simulink model "case1"  (R2024b)
settings: Solver=FixedStepAuto  StartTime=0  StopTime=1  FixedStep=1e-7  RelTol=1e-3
values from neighbouring files (symbols this model uses):
  SG_D_1_D = 0.01056    [IEEE9_case_parameters.m]    (also in case1_parameters.m; case2_parameters.m; case3_parameters.m; case4_parameters.m)
  SG_D_1_EnableSaturation = 0    [IEEE9_case_parameters.m]    (also in case1_parameters.m; case2_parameters.m; case3_parameters.m; case4_parameters.m)
  SG_D_1_f0 = 60    [IEEE9_case_parameters.m]    (also in case1_parameters.m; case2_parameters.m; case3_parameters.m; case4_parameters.m)
  SG_D_1_H = 7.5    [IEEE9_case_parameters.m]    (also in case1_parameters.m; case2_parameters.m; case3_parameters.m; case4_parameters.m)
  SG_D_1_K_A = 20    [IEEE9_case_parameters.m]    (also in case1_parameters.m; case2_parameters.m; case3_parameters.m; case4_parameters.m)
  SG_D_1_K_E = 1.000000e+1    (= 10)    [IEEE9_case_parameters.m]    (also in case1_parameters.m; case2_parameters.m; case3_parameters.m; case4_parameters.m)
  SG_D_1_K_F = 2.363    [IEEE9_case_parameters.m]    (also in case1_parameters.m; case2_parameters.m; case3_parameters.m; case4_parameters.m)
  SG_D_1_K_s = 0.5    [IEEE9_case_parameters.m]    (also in case1_parameters.m = 5; case2_parameters.m = 5; case3_parameters.m = 5; case4_parameters.m = 5)
  SG_D_1_R_a = 0.001088    [IEEE9_case_parameters.m]    (also in case1_parameters.m; case2_parameters.m; case3_parameters.m; case4_parameters.m)
  SG_D_1_S_A = 1    [IEEE9_case_parameters.m]    (also in case1_parameters.m; case2_parameters.m; case3_parameters.m; case4_parameters.m)
  SG_D_1_S_B = 0.103    [IEEE9_case_parameters.m]    (also in case1_parameters.m; case2_parameters.m; case3_parameters.m; case4_parameters.m)
  SG_D_1_S_N = 10.659857    [IEEE9_case_parameters.m]    (also in case1_parameters.m; case2_parameters.m; case3_parameters.m; case4_parameters.m)
  SG_D_1_SpeedPara = 200    [IEEE9_case_parameters.m]    (also in case1_parameters.m; case2_parameters.m; case3_parameters.m; case4_parameters.m)
  SG_D_1_T_0 = 0.720173    [IEEE9_case_parameters.m]    (also in case1_parameters.m = 0.755522; case2_parameters.m = 0.808931; case3_parameters.m = 0.869402; case4_parameters.m = 0.729316)
  SG_D_1_T_1 = 0.3    [IEEE9_case_parameters.m]    (also in case1_parameters.m; case2_parameters.m; case3_parameters.m; case4_parameters.m)
  SG_D_1_T_2 = 0.05    [IEEE9_case_parameters.m]    (also in case1_parameters.m; case2_parameters.m; case3_parameters.m; case4_parameters.m)
  SG_D_1_T_3 = 0.02    [IEEE9_case_parameters.m]    (also in case1_parameters.m; case2_parameters.m; case3_parameters.m; case4_parameters.m)
  SG_D_1_T_4 = 0.005    [IEEE9_case_parameters.m]    (also in case1_parameters.m; case2_parameters.m; case3_parameters.m; case4_parameters.m)
  SG_D_1_T_A = 0.02    [IEEE9_case_parameters.m]    (also in case1_parameters.m; case2_parameters.m; case3_parameters.m; case4_parameters.m)
  SG_D_1_T_dd = 8.000000e+0    (= 8)    [IEEE9_case_parameters.m]    (also in case1_parameters.m; case2_parameters.m; case3_parameters.m; case4_parameters.m)
  SG_D_1_T_ddd = 0.04    [IEEE9_case_parameters.m]    (also in case1_parameters.m; case2_parameters.m; case3_parameters.m; case4_parameters.m)
  SG_D_1_T_E = 0.314    [IEEE9_case_parameters.m]    (also in case1_parameters.m; case2_parameters.m; case3_parameters.m; case4_parameters.m)
  SG_D_1_T_F = 0.35    [IEEE9_case_parameters.m]    (also in case1_parameters.m; case2_parameters.m; case3_parameters.m; case4_parameters.m)
  SG_D_1_T_qd = 0.8    [IEEE9_case_parameters.m]    (also in case1_parameters.m; case2_parameters.m; case3_parameters.m; case4_parameters.m)
  SG_D_1_T_qdd = 0.02    [IEEE9_case_parameters.m]    (also in case1_parameters.m; case2_parameters.m; case3_parameters.m; case4_parameters.m)
  SG_D_1_T_speed = 0.1    [IEEE9_case_parameters.m]    (also in case1_parameters.m = 200; case2_parameters.m = 200; case3_parameters.m = 200; case4_parameters.m = 200)
  SG_D_1_T_w = 0.5    [IEEE9_case_parameters.m]    (also in case1_parameters.m; case2_parameters.m; case3_parameters.m; case4_parameters.m)
  SG_D_1_V_ref = 1.990276    [IEEE9_case_parameters.m]    (also in case1_parameters.m = 2.042296; case2_parameters.m = 2.051388; case3_parameters.m = 2.089584; case4_parameters.m = 2.01845)
  SG_D_1_w_ref = 376.991118    [IEEE9_case_parameters.m]    (also in case1_parameters.m; case2_parameters.m; case3_parameters.m; case4_parameters.m)
  SG_D_1_wb = 6.000000e+1    (= 60)    [IEEE9_case_parameters.m]    (also in case1_parameters.m; case2_parameters.m; case3_parameters.m; case4_parameters.m)
  SG_D_1_x_d = 1.9    [IEEE9_case_parameters.m]    (also in case1_parameters.m; case2_parameters.m; case3_parameters.m; case4_parameters.m)
  SG_D_1_x_dd = 0.302    [IEEE9_case_parameters.m]    (also in case1_parameters.m; case2_parameters.m; case3_parameters.m; case4_parameters.m)
  SG_D_1_x_ddd = 0.204    [IEEE9_case_parameters.m]    (also in case1_parameters.m; case2_parameters.m; case3_parameters.m; case4_parameters.m)
  SG_D_1_x_l = 0.05    [IEEE9_case_parameters.m]    (also in case1_parameters.m; case2_parameters.m; case3_parameters.m; case4_parameters.m)
  SG_D_1_x_q = 1.3    [IEEE9_case_parameters.m]    (also in case1_parameters.m; case2_parameters.m; case3_parameters.m; case4_parameters.m)
  SG_D_1_x_qd = 0.5    [IEEE9_case_parameters.m]    (also in case1_parameters.m; case2_parameters.m; case3_parameters.m; case4_parameters.m)
  SG_D_1_x_qdd = 0.3    [IEEE9_case_parameters.m]    (also in case1_parameters.m; case2_parameters.m; case3_parameters.m; case4_parameters.m)
  SG_D_2_D = 0.02    [IEEE9_case_parameters.m]    (also in case1_parameters.m; case2_parameters.m; case3_parameters.m; case4_parameters.m)
  SG_D_2_EnableSaturation = 0    [IEEE9_case_parameters.m]    (also in case1_parameters.m; case2_parameters.m; case3_parameters.m; case4_parameters.m)
  SG_D_2_f0 = 60    [IEEE9_case_parameters.m]    (also in case1_parameters.m; case2_parameters.m; case3_parameters.m; case4_parameters.m)
  SG_D_2_H = 8.000000e+0    (= 8)    [IEEE9_case_parameters.m]    (also in case1_parameters.m; case2_parameters.m; case3_parameters.m; case4_parameters.m)
  SG_D_2_K_A = 20    [IEEE9_case_parameters.m]    (also in case1_parameters.m; case2_parameters.m; case3_parameters.m; case4_parameters.m)
  SG_D_2_K_E = 1.000000e+1    (= 10)    [IEEE9_case_parameters.m]    (also in case1_parameters.m; case2_parameters.m; case3_parameters.m; case4_parameters.m)
  SG_D_2_K_F = 2.363    [IEEE9_case_parameters.m]    (also in case1_parameters.m; case2_parameters.m; case3_parameters.m; case4_parameters.m)
  SG_D_2_K_s = 0.5    [IEEE9_case_parameters.m]    (also in case1_parameters.m = 4; case2_parameters.m = 4; case3_parameters.m = 4; case4_parameters.m = 4)
  SG_D_2_R_a = 0.001088    [IEEE9_case_parameters.m]    (also in case1_parameters.m; case2_parameters.m; case3_parameters.m; case4_parameters.m)
  SG_D_2_S_A = 1    [IEEE9_case_parameters.m]    (also in case1_parameters.m; case2_parameters.m; case3_parameters.m; case4_parameters.m)
  SG_D_2_S_B = 0.103    [IEEE9_case_parameters.m]    (also in case1_parameters.m; case2_parameters.m; case3_parameters.m; case4_parameters.m)
  SG_D_2_S_N = 10.659857    [IEEE9_case_parameters.m]    (also in case1_parameters.m; case2_parameters.m; case3_parameters.m; case4_parameters.m)
  SG_D_2_SpeedPara = 200    [IEEE9_case_parameters.m]    (also in case1_parameters.m; case2_parameters.m; case3_parameters.m; case4_parameters.m)
  SG_D_2_T_0 = 1.632913    [IEEE9_case_parameters.m]    (also in case1_parameters.m = 1.632925; case2_parameters.m = 1.632915; case3_parameters.m = 1.632914; case4_parameters.m = 1.632927)
  SG_D_2_T_1 = 0.2    [IEEE9_case_parameters.m]    (also in case1_parameters.m; case2_parameters.m; case3_parameters.m; case4_parameters.m)
  SG_D_2_T_2 = 0.05    [IEEE9_case_parameters.m]    (also in case1_parameters.m; case2_parameters.m; case3_parameters.m; case4_parameters.m)
  SG_D_2_T_3 = 0.02    [IEEE9_case_parameters.m]    (also in case1_parameters.m; case2_parameters.m; case3_parameters.m; case4_parameters.m)
  SG_D_2_T_4 = 0.005    [IEEE9_case_parameters.m]    (also in case1_parameters.m; case2_parameters.m; case3_parameters.m; case4_parameters.m)
  SG_D_2_T_A = 0.02    [IEEE9_case_parameters.m]    (also in case1_parameters.m; case2_parameters.m; case3_parameters.m; case4_parameters.m)
  SG_D_2_T_dd = 7.9    [IEEE9_case_parameters.m]    (also in case1_parameters.m; case2_parameters.m; case3_parameters.m; case4_parameters.m)
  SG_D_2_T_ddd = 0.04    [IEEE9_case_parameters.m]    (also in case1_parameters.m; case2_parameters.m; case3_parameters.m; case4_parameters.m)
  SG_D_2_T_E = 0.314    [IEEE9_case_parameters.m]    (also in case1_parameters.m; case2_parameters.m; case3_parameters.m; case4_parameters.m)
  SG_D_2_T_F = 0.35    [IEEE9_case_parameters.m]    (also in case1_parameters.m; case2_parameters.m; case3_parameters.m; case4_parameters.m)
  SG_D_2_T_qd = 0.8    [IEEE9_case_parameters.m]    (also in case1_parameters.m; case2_parameters.m; case3_parameters.m; case4_parameters.m)
  SG_D_2_T_qdd = 0.015    [IEEE9_case_parameters.m]    (also in case1_parameters.m; case2_parameters.m; case3_parameters.m; case4_parameters.m)
  SG_D_2_T_speed = 0.1    [IEEE9_case_parameters.m]    (also in case1_parameters.m = 150; case2_parameters.m = 150; case3_parameters.m = 150; case4_parameters.m = 150)
  SG_D_2_T_w = 0.35    [IEEE9_case_parameters.m]    (also in case1_parameters.m; case2_parameters.m; case3_parameters.m; case4_parameters.m)
  SG_D_2_V_ref = 2.58547    [IEEE9_case_parameters.m]    (also in case1_parameters.m = 2.597896; case2_parameters.m = 2.587136; case3_parameters.m = 2.586042; case4_parameters.m = 2.599679)
  SG_D_2_w_ref = 376.991118    [IEEE9_case_parameters.m]    (also in case1_parameters.m; case2_parameters.m; case3_parameters.m; case4_parameters.m)
  SG_D_2_wb = 6.000000e+1    (= 60)    [IEEE9_case_parameters.m]    (also in case1_parameters.m; case2_parameters.m; case3_parameters.m; case4_parameters.m)
  SG_D_2_x_d = 1.8    [IEEE9_case_parameters.m]    (also in case1_parameters.m; case2_parameters.m; case3_parameters.m; case4_parameters.m)
  SG_D_2_x_dd = 0.302    [IEEE9_case_parameters.m]    (also in case1_parameters.m; case2_parameters.m; case3_parameters.m; case4_parameters.m)
  SG_D_2_x_ddd = 0.204    [IEEE9_case_parameters.m]    (also in case1_parameters.m; case2_parameters.m; case3_parameters.m; case4_parameters.m)
  SG_D_2_x_l = 0.05    [IEEE9_case_parameters.m]    (also in case1_parameters.m; case2_parameters.m; case3_parameters.m; case4_parameters.m)
  SG_D_2_x_q = 1.25    [IEEE9_case_parameters.m]    (also in case1_parameters.m; case2_parameters.m; case3_parameters.m; case4_parameters.m)
  SG_D_2_x_qd = 0.5    [IEEE9_case_parameters.m]    (also in case1_parameters.m; case2_parameters.m; case3_parameters.m; case4_parameters.m)
  SG_D_2_x_qdd = 0.3    [IEEE9_case_parameters.m]    (also in case1_parameters.m; case2_parameters.m; case3_parameters.m; case4_parameters.m)
  SG_D_3_D = 0.02    [IEEE9_case_parameters.m]    (also in case1_parameters.m; case2_parameters.m; case3_parameters.m; case4_parameters.m)
  SG_D_3_EnableSaturation = 0    [IEEE9_case_parameters.m]    (also in case1_parameters.m; case2_parameters.m; case3_parameters.m; case4_parameters.m)
  SG_D_3_f0 = 60    [IEEE9_case_parameters.m]    (also in case1_parameters.m; case2_parameters.m; case3_parameters.m; case4_parameters.m)
  SG_D_3_H = 7.7    [IEEE9_case_parameters.m]    (also in case1_parameters.m; case2_parameters.m; case3_parameters.m; case4_parameters.m)
  SG_D_3_K_A = 20    [IEEE9_case_parameters.m]    (also in case1_parameters.m; case2_parameters.m; case3_parameters.m; case4_parameters.m)
  SG_D_3_K_E = 1.000000e+1    (= 10)    [IEEE9_case_parameters.m]    (also in case1_parameters.m; case2_parameters.m; case3_parameters.m; case4_parameters.m)
  SG_D_3_K_F = 2.363    [IEEE9_case_parameters.m]    (also in case1_parameters.m; case2_parameters.m; case3_parameters.m; case4_parameters.m)
  SG_D_3_K_s = 0.2    [IEEE9_case_parameters.m]    (also in case1_parameters.m = 2; case2_parameters.m = 2; case3_parameters.m = 2; case4_parameters.m = 2)
  SG_D_3_R_a = 0.001088    [IEEE9_case_parameters.m]    (also in case1_parameters.m; case2_parameters.m; case3_parameters.m; case4_parameters.m)
  SG_D_3_S_A = 1    [IEEE9_case_parameters.m]    (also in case1_parameters.m; case2_parameters.m; case3_parameters.m; case4_parameters.m)
  SG_D_3_S_B = 0.103    [IEEE9_case_parameters.m]    (also in case1_parameters.m; case2_parameters.m; case3_parameters.m; case4_parameters.m)
  SG_D_3_S_N = 10.659857    [IEEE9_case_parameters.m]    (also in case1_parameters.m; case2_parameters.m; case3_parameters.m; case4_parameters.m)
  SG_D_3_SpeedPara = 200    [IEEE9_case_parameters.m]    (also in case1_parameters.m; case2_parameters.m; case3_parameters.m; case4_parameters.m)
  SG_D_3_T_0 = 0.850788    [IEEE9_case_parameters.m]    (also in case1_parameters.m = 0.850786; case2_parameters.m = 0.850787; case3_parameters.m; case4_parameters.m = 0.850786)
  SG_D_3_T_1 = 0.2    [IEEE9_case_parameters.m]    (also in case1_parameters.m; case2_parameters.m; case3_parameters.m; case4_parameters.m)
  SG_D_3_T_2 = 0.05    [IEEE9_case_parameters.m]    (also in case1_parameters.m; case2_parameters.m; case3_parameters.m; case4_parameters.m)
  SG_D_3_T_3 = 0.02    [IEEE9_case_parameters.m]    (also in case1_parameters.m; case2_parameters.m; case3_parameters.m; case4_parameters.m)
  SG_D_3_T_4 = 0.005    [IEEE9_case_parameters.m]    (also in case1_parameters.m; case2_parameters.m; case3_parameters.m; case4_parameters.m)
  SG_D_3_T_A = 0.02    [IEEE9_case_parameters.m]    (also in case1_parameters.m; case2_parameters.m; case3_parameters.m; case4_parameters.m)
  SG_D_3_T_dd = 8.1    [IEEE9_case_parameters.m]    (also in case1_parameters.m; case2_parameters.m; case3_parameters.m; case4_parameters.m)
  SG_D_3_T_ddd = 0.04    [IEEE9_case_parameters.m]    (also in case1_parameters.m; case2_parameters.m; case3_parameters.m; case4_parameters.m)
  SG_D_3_T_E = 0.314    [IEEE9_case_parameters.m]    (also in case1_parameters.m; case2_parameters.m; case3_parameters.m; case4_parameters.m)
  SG_D_3_T_F = 0.35    [IEEE9_case_parameters.m]    (also in case1_parameters.m; case2_parameters.m; case3_parameters.m; case4_parameters.m)
  SG_D_3_T_qd = 0.8    [IEEE9_case_parameters.m]    (also in case1_parameters.m; case2_parameters.m; case3_parameters.m; case4_parameters.m)
  SG_D_3_T_qdd = 0.015    [IEEE9_case_parameters.m]    (also in case1_parameters.m; case2_parameters.m; case3_parameters.m; case4_parameters.m)
  SG_D_3_T_speed = 0.1    [IEEE9_case_parameters.m]    (also in case1_parameters.m = 180; case2_parameters.m = 180; case3_parameters.m = 180; case4_parameters.m = 180)
  SG_D_3_T_w = 0.4    [IEEE9_case_parameters.m]    (also in case1_parameters.m; case2_parameters.m; case3_parameters.m; case4_parameters.m)
  SG_D_3_V_ref = 1.892727    [IEEE9_case_parameters.m]    (also in case1_parameters.m = 1.906439; case2_parameters.m = 1.895535; case3_parameters.m = 1.892105; case4_parameters.m = 1.906598)
  SG_D_3_w_ref = 376.991118    [IEEE9_case_parameters.m]    (also in case1_parameters.m; case2_parameters.m; case3_parameters.m; case4_parameters.m)
  SG_D_3_wb = 6.000000e+1    (= 60)    [IEEE9_case_parameters.m]    (also in case1_parameters.m; case2_parameters.m; case3_parameters.m; case4_parameters.m)
  SG_D_3_x_d = 1.85    [IEEE9_case_parameters.m]    (also in case1_parameters.m; case2_parameters.m; case3_parameters.m; case4_parameters.m)
  SG_D_3_x_dd = 0.302    [IEEE9_case_parameters.m]    (also in case1_parameters.m; case2_parameters.m; case3_parameters.m; case4_parameters.m)
  SG_D_3_x_ddd = 0.204    [IEEE9_case_parameters.m]    (also in case1_parameters.m; case2_parameters.m; case3_parameters.m; case4_parameters.m)
  SG_D_3_x_l = 0.05    [IEEE9_case_parameters.m]    (also in case1_parameters.m; case2_parameters.m; case3_parameters.m; case4_parameters.m)
  SG_D_3_x_q = 1.2    [IEEE9_case_parameters.m]    (also in case1_parameters.m; case2_parameters.m; case3_parameters.m; case4_parameters.m)
  SG_D_3_x_qd = 0.5    [IEEE9_case_parameters.m]    (also in case1_parameters.m; case2_parameters.m; case3_parameters.m; case4_parameters.m)
  SG_D_3_x_qdd = 0.3    [IEEE9_case_parameters.m]    (also in case1_parameters.m; case2_parameters.m; case3_parameters.m; case4_parameters.m)
(part 1 of 12)
settings Model: Creator=Greg  LastModifiedBy=Greg

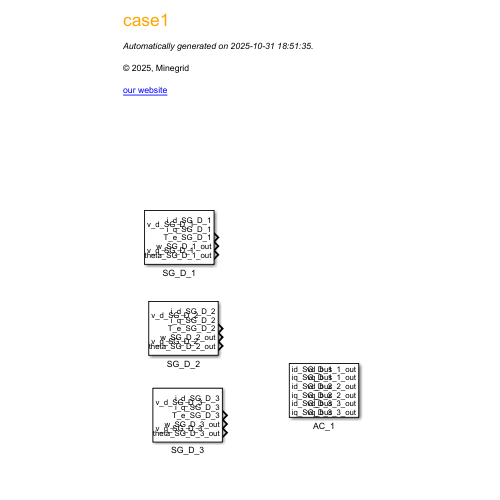
[thumbnail: Simulink's stored preview of the top-level diagram]
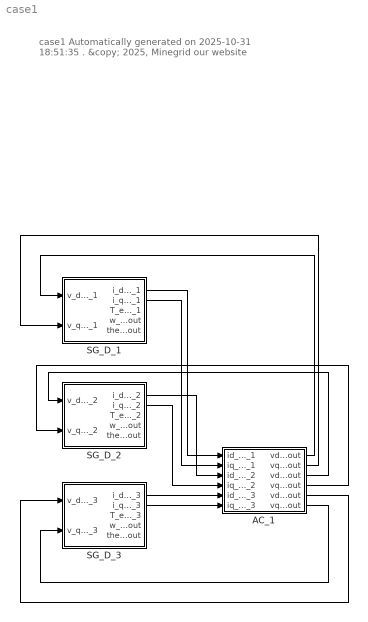
== system case1 ==
  note: case1
      | Automatically generated on 2025-10-31 18:51:35 .
      | &copy; 2025, Minegrid
      | our website
  AC_1 : Subsystem  mask(AC_1){}
      mask help: Parameters Interface of AC_1
  SG_D_1 : Subsystem  mask(SG_D_1){T_0=SG_D_1_T_0, w_ref=SG_D_1_w_ref, V_ref=SG_D_1_V_ref, x_d=SG_D_1_x_d, x_dd=SG_D_1_x_dd, x_ddd=SG_D_1_x_ddd, x_q=SG_D_1_x_q, x_qd=SG_D_1_x_qd, x_qdd=SG_D_1_x_qdd, x_l=SG_D_1_x_l, R_a=SG_D_1_R_a, T_dd=SG_D_1_T_dd, T_ddd=SG_D_1_T_ddd, T_qd=SG_D_1_T_qd, T_qdd=SG_D_1_T_qdd, H=SG_D_1_H, D=SG_D_1_D, SpeedPara=SG_D_1_SpeedPara, K_A=SG_D_1_K_A, EnableSaturation=SG_D_1_EnableSaturation, f0=SG_D_1_f0, T_speed=SG_D_1_T_speed, T_E=SG_D_1_T_E, T_A=SG_D_1_T_A, T_F=SG_D_1_T_F, K_E=SG_D_1_K_E, K_F=SG_D_1_K_F, K_s=SG_D_1_K_s, T_1=SG_D_1_T_1, T_2=SG_D_1_T_2, T_3=SG_D_1_T_3, T_4=SG_D_1_T_4, T_w=SG_D_1_T_w, wb=SG_D_1_wb, S_A=SG_D_1_S_A, S_B=SG_D_1_S_B, S_N=SG_D_1_S_N}
      mask help: Parameters Interface of SG_D_1
  SG_D_2 : Subsystem  mask(SG_D_2){T_0=SG_D_2_T_0, w_ref=SG_D_2_w_ref, V_ref=SG_D_2_V_ref, x_d=SG_D_2_x_d, x_dd=SG_D_2_x_dd, x_ddd=SG_D_2_x_ddd, x_q=SG_D_2_x_q, x_qd=SG_D_2_x_qd, x_qdd=SG_D_2_x_qdd, x_l=SG_D_2_x_l, R_a=SG_D_2_R_a, T_dd=SG_D_2_T_dd, T_ddd=SG_D_2_T_ddd, T_qd=SG_D_2_T_qd, T_qdd=SG_D_2_T_qdd, H=SG_D_2_H, D=SG_D_2_D, SpeedPara=SG_D_2_SpeedPara, K_A=SG_D_2_K_A, EnableSaturation=SG_D_2_EnableSaturation, f0=SG_D_2_f0, T_speed=SG_D_2_T_speed, T_E=SG_D_2_T_E, T_A=SG_D_2_T_A, T_F=SG_D_2_T_F, K_E=SG_D_2_K_E, K_F=SG_D_2_K_F, K_s=SG_D_2_K_s, T_1=SG_D_2_T_1, T_2=SG_D_2_T_2, T_3=SG_D_2_T_3, T_4=SG_D_2_T_4, T_w=SG_D_2_T_w, wb=SG_D_2_wb, S_A=SG_D_2_S_A, S_B=SG_D_2_S_B, S_N=SG_D_2_S_N}
      mask help: Parameters Interface of SG_D_2
  SG_D_3 : Subsystem  mask(SG_D_3){T_0=SG_D_3_T_0, w_ref=SG_D_3_w_ref, V_ref=SG_D_3_V_ref, x_d=SG_D_3_x_d, x_dd=SG_D_3_x_dd, x_ddd=SG_D_3_x_ddd, x_q=SG_D_3_x_q, x_qd=SG_D_3_x_qd, x_qdd=SG_D_3_x_qdd, x_l=SG_D_3_x_l, R_a=SG_D_3_R_a, T_dd=SG_D_3_T_dd, T_ddd=SG_D_3_T_ddd, T_qd=SG_D_3_T_qd, T_qdd=SG_D_3_T_qdd, H=SG_D_3_H, D=SG_D_3_D, SpeedPara=SG_D_3_SpeedPara, K_A=SG_D_3_K_A, EnableSaturation=SG_D_3_EnableSaturation, f0=SG_D_3_f0, T_speed=SG_D_3_T_speed, T_E=SG_D_3_T_E, T_A=SG_D_3_T_A, T_F=SG_D_3_T_F, K_E=SG_D_3_K_E, K_F=SG_D_3_K_F, K_s=SG_D_3_K_s, T_1=SG_D_3_T_1, T_2=SG_D_3_T_2, T_3=SG_D_3_T_3, T_4=SG_D_3_T_4, T_w=SG_D_3_T_w, wb=SG_D_3_wb, S_A=SG_D_3_S_A, S_B=SG_D_3_S_B, S_N=SG_D_3_S_N}
      mask help: Parameters Interface of SG_D_3
  wires:
  SG_D_2/2(i_q_SG_D_2) -> AC_1/4(iq_SG_D_2)
  SG_D_1/2(i_q_SG_D_1) -> AC_1/2(iq_SG_D_1)
  SG_D_1/1(i_d_SG_D_1) -> AC_1/1(id_SG_D_1)
  SG_D_2/1(i_d_SG_D_2) -> AC_1/3(id_SG_D_2)
  AC_1/1(vd_bus_1_out) -> SG_D_1/1(v_d_SG_D_1)
  SG_D_3/1(i_d_SG_D_3) -> AC_1/5(id_SG_D_3)
  AC_1/2(vq_bus_1_out) -> SG_D_1/2(v_q_SG_D_1)
  SG_D_3/2(i_q_SG_D_3) -> AC_1/6(iq_SG_D_3)
  AC_1/3(vd_bus_2_out) -> SG_D_2/1(v_d_SG_D_2)
  AC_1/4(vq_bus_2_out) -> SG_D_2/2(v_q_SG_D_2)
  AC_1/5(vd_bus_3_out) -> SG_D_3/1(v_d_SG_D_3)
  AC_1/6(vq_bus_3_out) -> SG_D_3/2(v_q_SG_D_3)

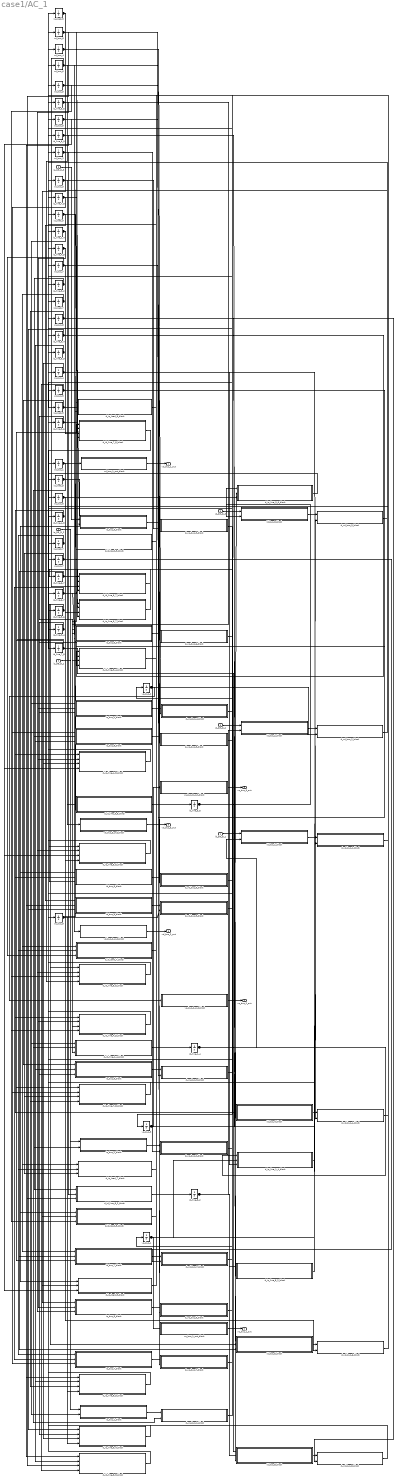
== system case1/AC_1 ==
  id_SG_D_1 : Inport
  iq_SG_D_1 : Inport  Port=2
  id_SG_D_2 : Inport  Port=3
  iq_SG_D_2 : Inport  Port=4
  id_SG_D_3 : Inport  Port=5
  iq_SG_D_3 : Inport  Port=6
  d_id_line_1_4_block : Subsystem
  d_id_line_3_6_block : Subsystem
  d_id_line_4_5_block : Subsystem
  d_id_line_5_6_block : Subsystem
  d_id_line_6_7_block : Subsystem
  d_id_line_7_8_block : Subsystem
  d_id_line_8_2_block : Subsystem
  d_id_line_8_9_block : Subsystem
  d_id_line_9_4_block : Subsystem
  d_id_load_5_block : Subsystem
  d_id_load_7_block : Subsystem
  d_id_load_9_block : Subsystem
  d_iq_line_1_4_block : Subsystem
  d_iq_line_3_6_block : Subsystem
  d_iq_line_4_5_block : Subsystem
  d_iq_line_5_6_block : Subsystem
  d_iq_line_6_7_block : Subsystem
  d_iq_line_7_8_block : Subsystem
  d_iq_line_8_2_block : Subsystem
  d_iq_line_8_9_block : Subsystem
  d_iq_line_9_4_block : Subsystem
  d_iq_load_5_block : Subsystem
  d_iq_load_7_block : Subsystem
  d_iq_load_9_block : Subsystem
  d_vd_bus_1_block : Subsystem
  d_vd_bus_2_block : Subsystem
  d_vd_bus_3_block : Subsystem
  d_vd_bus_4_block : Subsystem
  d_vd_bus_5_block : Subsystem
  d_vd_bus_6_block : Subsystem
  d_vd_bus_7_block : Subsystem
  d_vd_bus_8_block : Subsystem
  d_vd_bus_9_block : Subsystem
  d_vq_bus_1_block : Subsystem
  d_vq_bus_2_block : Subsystem
  d_vq_bus_3_block : Subsystem
  d_vq_bus_4_block : Subsystem
  d_vq_bus_5_block : Subsystem
  d_vq_bus_6_block : Subsystem
  d_vq_bus_7_block : Subsystem
  d_vq_bus_8_block : Subsystem
  d_vq_bus_9_block : Subsystem
  id_bus_1_block : Subsystem
  id_bus_2_block : Subsystem
  id_bus_3_block : Subsystem
  id_bus_4_block : Subsystem
  id_bus_5_block : Subsystem
  id_bus_6_block : Subsystem
  id_bus_7_block : Subsystem
  id_bus_8_block : Subsystem
  id_bus_9_block : Subsystem
  id_line_1_4 : Integrator  InitialCondition=0.7548
  id_line_3_6 : Integrator  InitialCondition=0.8464
  id_line_4_5 : Integrator  InitialCondition=0.3237
  id_line_5_6 : Integrator  InitialCondition=-0.6042
  id_line_6_7 : Integrator  InitialCondition=0.2507
  id_line_7_8 : Integrator  InitialCondition=-0.7792
  id_line_8_2 : Integrator  InitialCondition=-1.6368
  id_line_8_9 : Integrator  InitialCondition=0.8719
  id_line_9_4 : Integrator  InitialCondition=-0.4237
  id_load_5 : Integrator  InitialCondition=0.9089751333440371
  id_load_7 : Integrator  InitialCondition=1.030922594542028
  id_load_9 : Integrator  InitialCondition=1.276894849415514
  iq_bus_1_block : Subsystem
  iq_bus_2_block : Subsystem
  iq_bus_3_block : Subsystem
  iq_bus_4_block : Subsystem
  iq_bus_5_block : Subsystem
  iq_bus_6_block : Subsystem
  iq_bus_7_block : Subsystem
  iq_bus_8_block : Subsystem
  iq_bus_9_block : Subsystem
  iq_line_1_4 : Integrator  InitialCondition=-0.2822
  iq_line_3_6 : Integrator  InitialCondition=0.0786
  iq_line_4_5 : Integrator  InitialCondition=-0.0984
  iq_line_5_6 : Integrator  InitialCondition=0.0494
  iq_line_6_7 : Integrator  InitialCondition=-0.156
  iq_line_7_8 : Integrator  InitialCondition=0.0401
  iq_line_8_2 : Integrator  InitialCondition=-0.0981
  iq_line_8_9 : Integrator  InitialCondition=-0.0875
  iq_line_9_4 : Integrator  InitialCondition=0.348
  iq_load_5 : Integrator  InitialCondition=-0.3975948941241939
  iq_load_7 : Integrator  InitialCondition=-0.37188300071282737
  iq_load_9 : Integrator  InitialCondition=-0.6641048777062669
  vd_bus_1 : Integrator  InitialCondition=1.0
  vd_bus_1_out_block : Subsystem
  vd_bus_2 : Integrator  InitialCondition=0.985803143460073
  vd_bus_2_out_block : Subsystem
  vd_bus_3 : Integrator  InitialCondition=0.9967347320434884
  vd_bus_3_out_block : Subsystem
  vd_bus_4 : Integrator  InitialCondition=0.9833478056182255
  vd_bus_5 : Integrator  InitialCondition=0.9683503471400442
  vd_bus_6 : Integrator  InitialCondition=1.0014525575970927
  vd_bus_7 : Integrator  InitialCondition=0.9822415146340815
  vd_bus_8 : Integrator  InitialCondition=0.9920858565379774
  vd_bus_9 : Integrator  InitialCondition=0.948636147702384
  vq_bus_1 : Integrator  InitialCondition=0.0
  vq_bus_1_out_block : Subsystem
  vq_bus_2 : Integrator  InitialCondition=0.16790521833534158
  vq_bus_2_out_block : Subsystem
  vq_bus_3 : Integrator  InitialCondition=0.08074573634685275
  vq_bus_3_out_block : Subsystem
  vq_bus_4 : Integrator  InitialCondition=-0.04454614993614489
  vq_bus_5 : Integrator  InitialCondition=-0.07331558532421262
  vq_bus_6 : Integrator  InitialCondition=0.029926298842353146
  vq_bus_7 : Integrator  InitialCondition=0.005967185456729667
  vq_bus_8 : Integrator  InitialCondition=0.0630927939475754
  vq_bus_9 : Integrator  InitialCondition=-0.07782842087829349
  vd_bus_1_out : Outport
  vq_bus_1_out : Outport  Port=2
  vd_bus_2_out : Outport  Port=3
  vq_bus_2_out : Outport  Port=4
  vd_bus_3_out : Outport  Port=5
  vq_bus_3_out : Outport  Port=6
  wires:
  d_id_line_9_4_block/1(Blockout_d_id_line_9_4_20edc) -> id_line_9_4/1
  vq_bus_5/1 -> d_iq_load_5_block/3(State_vq_bus_5_2f3a6), d_iq_line_5_6_block/3(State_vq_bus_5_b22ab), d_iq_line_4_5_block/4(State_vq_bus_5_04a69), d_vd_bus_5_block/2(State_vq_bus_5_226eb)
  iq_SG_D_1/1 -> iq_bus_1_block/1(Input_iq_SG_D_1_6fe57)
  id_bus_9_block/1(Blockout_id_bus_9_d8517) -> d_vd_bus_9_block/1(Alge_id_bus_9_1ac5c)
  vq_bus_2_out_block/1(Blockout_vq_bus_2_out_5caa2) -> vq_bus_2_out/1
  d_id_line_1_4_block/1(Blockout_d_id_line_1_4_02e23) -> id_line_1_4/1
  iq_SG_D_3/1 -> iq_bus_3_block/1(Input_iq_SG_D_3_98297)
  d_vd_bus_7_block/1(Blockout_d_vd_bus_7_eeed9) -> vd_bus_7/1
  id_bus_8_block/1(Blockout_id_bus_8_9838c) -> d_vd_bus_8_block/1(Alge_id_bus_8_bb1f2)
  id_bus_3_block/1(Blockout_id_bus_3_3aea8) -> d_vd_bus_3_block/1(Alge_id_bus_3_b8f2d)
  vd_bus_5/1 -> d_vq_bus_5_block/2(State_vd_bus_5_1574f), d_id_line_5_6_block/3(State_vd_bus_5_4803e), d_id_load_5_block/3(State_vd_bus_5_1aa4f), d_id_line_4_5_block/4(State_vd_bus_5_d1c47)
  d_iq_line_5_6_block/1(Blockout_d_iq_line_5_6_8d1bb) -> iq_line_5_6/1
  iq_line_6_7/1 -> d_id_line_6_7_block/2(State_iq_line_6_7_9688a), d_iq_line_6_7_block/2(State_iq_line_6_7_6494b), iq_bus_6_block/3(State_iq_line_6_7_100bb), iq_bus_7_block/2(State_iq_line_6_7_6bc6f)
  iq_line_7_8/1 -> d_id_line_7_8_block/2(State_iq_line_7_8_d3a92), iq_bus_8_block/1(State_iq_line_7_8_4bd2e), d_iq_line_7_8_block/2(State_iq_line_7_8_50859), iq_bus_7_block/3(State_iq_line_7_8_d005c)
  d_iq_line_8_2_block/1(Blockout_d_iq_line_8_2_543a1) -> iq_line_8_2/1
  id_SG_D_3/1 -> id_bus_3_block/1(Input_id_SG_D_3_c7560)
  d_vd_bus_4_block/1(Blockout_d_vd_bus_4_c0860) -> vd_bus_4/1
  vd_bus_3_out_block/1(Blockout_vd_bus_3_out_e6f06) -> vd_bus_3_out/1
  iq_SG_D_2/1 -> iq_bus_2_block/1(Input_iq_SG_D_2_5d5eb)
  vq_bus_2/1 -> d_vd_bus_2_block/2(State_vq_bus_2_b534c), d_iq_line_8_2_block/2(State_vq_bus_2_eedb1), vq_bus_2_out_block/1(State_vq_bus_2_101ce)
  id_SG_D_2/1 -> id_bus_2_block/1(Input_id_SG_D_2_52bf0)
  iq_bus_1_block/1(Blockout_iq_bus_1_a9d09) -> d_vq_bus_1_block/1(Alge_iq_bus_1_aaaa9)
  id_SG_D_1/1 -> id_bus_1_block/1(Input_id_SG_D_1_23990)
  d_iq_load_7_block/1(Blockout_d_iq_load_7_2f8c2) -> iq_load_7/1
  id_line_7_8/1 -> id_bus_8_block/1(State_id_line_7_8_3ae3c), id_bus_7_block/3(State_id_line_7_8_5b752), d_id_line_7_8_block/1(State_id_line_7_8_8dd6f), d_iq_line_7_8_block/1(State_id_line_7_8_27216)
  id_line_6_7/1 -> id_bus_6_block/3(State_id_line_6_7_bc3d2), d_id_line_6_7_block/1(State_id_line_6_7_fdc4e), d_iq_line_6_7_block/1(State_id_line_6_7_d6333), id_bus_7_block/2(State_id_line_6_7_ab1bc)
  id_bus_2_block/1(Blockout_id_bus_2_bdcc8) -> d_vd_bus_2_block/1(Alge_id_bus_2_38876)
  iq_bus_4_block/1(Blockout_iq_bus_4_f7785) -> d_vq_bus_4_block/1(Alge_iq_bus_4_eaffa)
  iq_bus_9_block/1(Blockout_iq_bus_9_07c34) -> d_vq_bus_9_block/1(Alge_iq_bus_9_ce7a0)
  vq_bus_3_out_block/1(Blockout_vq_bus_3_out_93aa3) -> vq_bus_3_out/1
  iq_bus_8_block/1(Blockout_iq_bus_8_1bc28) -> d_vq_bus_8_block/1(Alge_iq_bus_8_dc6f7)
  d_id_load_5_block/1(Blockout_d_id_load_5_7c560) -> id_load_5/1
  iq_bus_5_block/1(Blockout_iq_bus_5_6e2a7) -> d_vq_bus_5_block/1(Alge_iq_bus_5_a9f44)
  d_id_line_8_2_block/1(Blockout_d_id_line_8_2_bde2e) -> id_line_8_2/1
  d_id_load_7_block/1(Blockout_d_id_load_7_3ab02) -> id_load_7/1
  iq_bus_6_block/1(Blockout_iq_bus_6_b8b39) -> d_vq_bus_6_block/1(Alge_iq_bus_6_2e2a2)
  d_vq_bus_2_block/1(Blockout_d_vq_bus_2_1031e) -> vq_bus_2/1
  id_bus_1_block/1(Blockout_id_bus_1_33f85) -> d_vd_bus_1_block/1(Alge_id_bus_1_738e1)
  id_line_1_4/1 -> d_iq_line_1_4_block/1(State_id_line_1_4_e2784), id_bus_4_block/1(State_id_line_1_4_58bbd), id_bus_1_block/2(State_id_line_1_4_dac35)
  iq_bus_7_block/1(Blockout_iq_bus_7_2e710) -> d_vq_bus_7_block/1(Alge_iq_bus_7_85db4)
  iq_load_7/1 -> d_id_load_7_block/2(State_iq_load_7_7baed), d_iq_load_7_block/2(State_iq_load_7_f715f), iq_bus_7_block/1(State_iq_load_7_b0e2f)
  id_bus_7_block/1(Blockout_id_bus_7_b6ff1) -> d_vd_bus_7_block/1(Alge_id_bus_7_e5b9f)
  id_line_4_5/1 -> id_bus_4_block/2(State_id_line_4_5_ac403), d_id_line_4_5_block/1(State_id_line_4_5_2f9d9), d_iq_line_4_5_block/1(State_id_line_4_5_305b5), id_bus_5_block/2(State_id_line_4_5_8dac8)
  id_bus_6_block/1(Blockout_id_bus_6_229a8) -> d_vd_bus_6_block/1(Alge_id_bus_6_1fc99)
  id_load_7/1 -> d_id_load_7_block/1(State_id_load_7_7e244), id_bus_7_block/1(State_id_load_7_eaed7), d_iq_load_7_block/1(State_id_load_7_47db6)
  id_bus_5_block/1(Blockout_id_bus_5_517a7) -> d_vd_bus_5_block/1(Alge_id_bus_5_af057)
  id_bus_4_block/1(Blockout_id_bus_4_e4a8c) -> d_vd_bus_4_block/1(Alge_id_bus_4_47562)
  vd_bus_1_out_block/1(Blockout_vd_bus_1_out_31117) -> vd_bus_1_out/1
  vq_bus_1_out_block/1(Blockout_vq_bus_1_out_f8f58) -> vq_bus_1_out/1
  vq_bus_7/1 -> d_vd_bus_7_block/2(State_vq_bus_7_885c9), d_iq_load_7_block/3(State_vq_bus_7_c9f78), d_iq_line_7_8_block/3(State_vq_bus_7_1c43c), d_iq_line_6_7_block/4(State_vq_bus_7_386f3)
  iq_load_9/1 -> d_id_load_9_block/2(State_iq_load_9_2b565), d_iq_load_9_block/2(State_iq_load_9_2bff1), iq_bus_9_block/1(State_iq_load_9_04094)
  id_load_5/1 -> d_id_load_5_block/1(State_id_load_5_a7934), id_bus_5_block/1(State_id_load_5_329c5), d_iq_load_5_block/1(State_id_load_5_781f5)
  iq_bus_3_block/1(Blockout_iq_bus_3_1800f) -> d_vq_bus_3_block/1(Alge_iq_bus_3_939b5)
  vd_bus_8/1 -> d_id_line_8_2_block/3(State_vd_bus_8_5928a), d_id_line_8_9_block/3(State_vd_bus_8_54a05), d_vq_bus_8_block/2(State_vd_bus_8_2280e), d_id_line_7_8_block/4(State_vd_bus_8_2c1e2)
  d_vd_bus_8_block/1(Blockout_d_vd_bus_8_835b6) -> vd_bus_8/1
  iq_bus_2_block/1(Blockout_iq_bus_2_a400f) -> d_vq_bus_2_block/1(Alge_iq_bus_2_d5b4f)
  vq_bus_8/1 -> d_iq_line_7_8_block/4(State_vq_bus_8_5c564), d_iq_line_8_9_block/3(State_vq_bus_8_6b472), d_vd_bus_8_block/2(State_vq_bus_8_682c6), d_iq_line_8_2_block/3(State_vq_bus_8_e41a9)
  id_line_9_4/1 -> id_bus_4_block/3(State_id_line_9_4_ed76d), d_iq_line_9_4_block/1(State_id_line_9_4_c7272), id_bus_9_block/3(State_id_line_9_4_85e6f), d_id_line_9_4_block/1(State_id_line_9_4_23399)
  d_id_load_9_block/1(Blockout_d_id_load_9_6afbf) -> id_load_9/1
  id_line_3_6/1 -> id_bus_3_block/2(State_id_line_3_6_bccaf), id_bus_6_block/1(State_id_line_3_6_274c1), d_iq_line_3_6_block/1(State_id_line_3_6_f913b)
  vd_bus_2_out_block/1(Blockout_vd_bus_2_out_8740e) -> vd_bus_2_out/1
  d_vq_bus_6_block/1(Blockout_d_vq_bus_6_1e8a2) -> vq_bus_6/1
  id_line_8_9/1 -> d_id_line_8_9_block/1(State_id_line_8_9_76f67), id_bus_8_block/3(State_id_line_8_9_9335c), id_bus_9_block/2(State_id_line_8_9_b8e8c), d_iq_line_8_9_block/1(State_id_line_8_9_64212)
  d_id_line_3_6_block/1(Blockout_d_id_line_3_6_44702) -> id_line_3_6/1
  vd_bus_1/1 -> d_vq_bus_1_block/2(State_vd_bus_1_fc5b3), vd_bus_1_out_block/1(State_vd_bus_1_cf04b), d_id_line_1_4_block/2(State_vd_bus_1_63720)
  iq_line_8_9/1 -> d_id_line_8_9_block/2(State_iq_line_8_9_c72f1), d_iq_line_8_9_block/2(State_iq_line_8_9_91aab), iq_bus_9_block/2(State_iq_line_8_9_2cb5f), iq_bus_8_block/3(State_iq_line_8_9_4f885)
  id_line_8_2/1 -> d_iq_line_8_2_block/1(State_id_line_8_2_17219), id_bus_8_block/2(State_id_line_8_2_8ae43), id_bus_2_block/2(State_id_line_8_2_e06f3)
  iq_line_9_4/1 -> d_id_line_9_4_block/2(State_iq_line_9_4_9f86a), d_iq_line_9_4_block/2(State_iq_line_9_4_4bacc), iq_bus_4_block/3(State_iq_line_9_4_b5c11), iq_bus_9_block/3(State_iq_line_9_4_7546b)
  vq_bus_9/1 -> d_iq_load_9_block/3(State_vq_bus_9_8e131), d_iq_line_8_9_block/4(State_vq_bus_9_3314f), d_iq_line_9_4_block/4(State_vq_bus_9_f6455), d_vd_bus_9_block/2(State_vq_bus_9_a5e2a)
  iq_line_8_2/1 -> d_id_line_8_2_block/1(State_iq_line_8_2_ef0f1), iq_bus_2_block/2(State_iq_line_8_2_b9f43), iq_bus_8_block/2(State_iq_line_8_2_22f52)
  id_line_5_6/1 -> d_id_line_5_6_block/1(State_id_line_5_6_678c2), d_iq_line_5_6_block/1(State_id_line_5_6_4698d), id_bus_5_block/3(State_id_line_5_6_8622f), id_bus_6_block/2(State_id_line_5_6_a25b6)
  iq_line_1_4/1 -> d_id_line_1_4_block/1(State_iq_line_1_4_1aaa5), iq_bus_4_block/1(State_iq_line_1_4_208ce), iq_bus_1_block/2(State_iq_line_1_4_19711)
  vq_bus_1/1 -> vq_bus_1_out_block/1(State_vq_bus_1_2880f), d_vd_bus_1_block/2(State_vq_bus_1_68a3e), d_iq_line_1_4_block/2(State_vq_bus_1_cc1a1)
  iq_line_4_5/1 -> d_id_line_4_5_block/2(State_iq_line_4_5_28448), iq_bus_4_block/2(State_iq_line_4_5_c03c7), iq_bus_5_block/2(State_iq_line_4_5_29371), d_iq_line_4_5_block/2(State_iq_line_4_5_0a9d2)
  vd_bus_9/1 -> d_vq_bus_9_block/2(State_vd_bus_9_7cb95), d_id_load_9_block/3(State_vd_bus_9_97729), d_id_line_9_4_block/4(State_vd_bus_9_43177), d_id_line_8_9_block/4(State_vd_bus_9_ba6dc)
  iq_line_3_6/1 -> d_id_line_3_6_block/1(State_iq_line_3_6_218be), iq_bus_3_block/2(State_iq_line_3_6_41bc5), iq_bus_6_block/1(State_iq_line_3_6_b594c)
  iq_line_5_6/1 -> d_id_line_5_6_block/2(State_iq_line_5_6_30e91), d_iq_line_5_6_block/2(State_iq_line_5_6_e5c27), iq_bus_5_block/3(State_iq_line_5_6_b096e), iq_bus_6_block/2(State_iq_line_5_6_ff608)
  vq_bus_4/1 -> d_iq_line_1_4_block/3(State_vq_bus_4_b95c1), d_iq_line_4_5_block/3(State_vq_bus_4_e89f1), d_iq_line_9_4_block/3(State_vq_bus_4_fd03e), d_vd_bus_4_block/2(State_vq_bus_4_5b78f)
  vd_bus_6/1 -> d_vq_bus_6_block/2(State_vd_bus_6_e07dd), d_id_line_5_6_block/4(State_vd_bus_6_fd499), d_id_line_3_6_block/3(State_vd_bus_6_af45e), d_id_line_6_7_block/3(State_vd_bus_6_febc2)
  id_load_9/1 -> d_id_load_9_block/1(State_id_load_9_6175e), d_iq_load_9_block/1(State_id_load_9_ebd3b), id_bus_9_block/1(State_id_load_9_d5952)
  iq_load_5/1 -> d_id_load_5_block/2(State_iq_load_5_1055a), d_iq_load_5_block/2(State_iq_load_5_1b8dc), iq_bus_5_block/1(State_iq_load_5_fd86e)
  vd_bus_7/1 -> d_vq_bus_7_block/2(State_vd_bus_7_89a44), d_id_load_7_block/3(State_vd_bus_7_6ff07), d_id_line_6_7_block/4(State_vd_bus_7_50435), d_id_line_7_8_block/3(State_vd_bus_7_5e09f)
  vd_bus_4/1 -> d_vq_bus_4_block/2(State_vd_bus_4_afc07), d_id_line_4_5_block/3(State_vd_bus_4_1e1bc), d_id_line_9_4_block/3(State_vd_bus_4_9315c), d_id_line_1_4_block/3(State_vd_bus_4_e2161)
  vd_bus_2/1 -> d_vq_bus_2_block/2(State_vd_bus_2_40a78), d_id_line_8_2_block/2(State_vd_bus_2_8c8c2), vd_bus_2_out_block/1(State_vd_bus_2_8d3e6)
  vq_bus_6/1 -> d_iq_line_3_6_block/3(State_vq_bus_6_03933), d_vd_bus_6_block/2(State_vq_bus_6_78a87), d_iq_line_5_6_block/4(State_vq_bus_6_bf656), d_iq_line_6_7_block/3(State_vq_bus_6_af623)
  vd_bus_3/1 -> d_vq_bus_3_block/2(State_vd_bus_3_ddba3), vd_bus_3_out_block/1(State_vd_bus_3_84175), d_id_line_3_6_block/2(State_vd_bus_3_5f170)
  vq_bus_3/1 -> d_vd_bus_3_block/2(State_vq_bus_3_2388c), d_iq_line_3_6_block/2(State_vq_bus_3_5a1c9), vq_bus_3_out_block/1(State_vq_bus_3_18347)
  d_id_line_5_6_block/1(Blockout_d_id_line_5_6_1f7ce) -> id_line_5_6/1
  d_iq_load_5_block/1(Blockout_d_iq_load_5_d2ff1) -> iq_load_5/1
  d_id_line_7_8_block/1(Blockout_d_id_line_7_8_4d2a9) -> id_line_7_8/1
  d_id_line_4_5_block/1(Blockout_d_id_line_4_5_a9a06) -> id_line_4_5/1
  d_vq_bus_8_block/1(Blockout_d_vq_bus_8_79652) -> vq_bus_8/1
  d_vd_bus_9_block/1(Blockout_d_vd_bus_9_2d149) -> vd_bus_9/1
  d_id_line_6_7_block/1(Blockout_d_id_line_6_7_4abc2) -> id_line_6_7/1
  d_id_line_8_9_block/1(Blockout_d_id_line_8_9_bdb89) -> id_line_8_9/1
  d_iq_line_1_4_block/1(Blockout_d_iq_line_1_4_78aac) -> iq_line_1_4/1
  d_iq_line_3_6_block/1(Blockout_d_iq_line_3_6_784c0) -> iq_line_3_6/1
  d_iq_line_4_5_block/1(Blockout_d_iq_line_4_5_e1e40) -> iq_line_4_5/1
  d_iq_line_6_7_block/1(Blockout_d_iq_line_6_7_6cbac) -> iq_line_6_7/1
  d_iq_line_7_8_block/1(Blockout_d_iq_line_7_8_28933) -> iq_line_7_8/1
  d_iq_line_8_9_block/1(Blockout_d_iq_line_8_9_f1949) -> iq_line_8_9/1
  d_vd_bus_3_block/1(Blockout_d_vd_bus_3_b64ce) -> vd_bus_3/1
  d_iq_line_9_4_block/1(Blockout_d_iq_line_9_4_f2aeb) -> iq_line_9_4/1
  d_vd_bus_1_block/1(Blockout_d_vd_bus_1_e1401) -> vd_bus_1/1
  d_iq_load_9_block/1(Blockout_d_iq_load_9_225bd) -> iq_load_9/1
  d_vd_bus_2_block/1(Blockout_d_vd_bus_2_81105) -> vd_bus_2/1
  d_vq_bus_3_block/1(Blockout_d_vq_bus_3_a043d) -> vq_bus_3/1
  d_vq_bus_1_block/1(Blockout_d_vq_bus_1_0a2d1) -> vq_bus_1/1
  d_vd_bus_5_block/1(Blockout_d_vd_bus_5_8fe13) -> vd_bus_5/1
  d_vd_bus_6_block/1(Blockout_d_vd_bus_6_d75a1) -> vd_bus_6/1
  d_vq_bus_4_block/1(Blockout_d_vq_bus_4_e20db) -> vq_bus_4/1
  d_vq_bus_5_block/1(Blockout_d_vq_bus_5_d5d5a) -> vq_bus_5/1
  d_vq_bus_7_block/1(Blockout_d_vq_bus_7_1fb71) -> vq_bus_7/1
  d_vq_bus_9_block/1(Blockout_d_vq_bus_9_cbc85) -> vq_bus_9/1

== system case1/SG_D_1 ==
  v_d_SG_D_1 : Inport
  v_q_SG_D_1 : Inport  Port=2
  E_fd_SG_D_1 : Integrator  InitialCondition=2.0845926160709487
  Px_1_SG_D_1 : Integrator  InitialCondition=0.0
  Px_2_SG_D_1 : Integrator  InitialCondition=0.0
  Px_3_SG_D_1 : Integrator  InitialCondition=6.149011643986097e-28
  R_f_SG_D_1 : Integrator  InitialCondition=14.073978147930434
  T_e_SG_D_1_block : Subsystem
  T_m_SG_D_1 : Integrator  InitialCondition=0.7555220859910107
  V_f_SG_D_1 : Integrator  InitialCondition=20.845926160709485
  d_E_fd_SG_D_1_block : Subsystem
  d_Px_1_SG_D_1_block : Subsystem
  d_Px_2_SG_D_1_block : Subsystem
  d_Px_3_SG_D_1_block : Subsystem
  d_R_f_SG_D_1_block : Subsystem
  d_T_m_SG_D_1_block : Subsystem
  d_V_f_SG_D_1_block : Subsystem
  d_psi_1d_SG_D_1_block : Subsystem
  d_psi_d_SG_D_1_block : Subsystem
  d_psi_fd_SG_D_1_block : Subsystem
  d_psi_gq_SG_D_1_block : Subsystem
  d_psi_kq_SG_D_1_block : Subsystem
  d_psi_q_SG_D_1_block : Subsystem
  d_theta_SG_D_1_block : Subsystem
  d_w_SG_D_1_block : Subsystem
  i_d_SG_D_1_block : Subsystem
  i_q_SG_D_1_block : Subsystem
  psi_1d_SG_D_1 : Integrator  InitialCondition=0.8465371880346609
  psi_d_SG_D_1 : Integrator  InitialCondition=0.8130762305201664
  psi_fd_SG_D_1 : Integrator  InitialCondition=1.015180413907712
  psi_gq_SG_D_1 : Integrator  InitialCondition=0.3591180733085622
  psi_kq_SG_D_1 : Integrator  InitialCondition=-0.5611219895446284
  psi_q_SG_D_1 : Integrator  InitialCondition=-0.5835668691264136
  theta_SG_D_1 : Integrator  InitialCondition=0.622217811004452
  theta_SG_D_1_out_block : Subsystem
  w_SG_D_1 : Integrator  InitialCondition=376.99111843077515
  w_SG_D_1_out_block : Subsystem
  i_d_SG_D_1 : Outport
  i_q_SG_D_1 : Outport  Port=2
  T_e_SG_D_1 : Outport  Port=3
  w_SG_D_1_out : Outport  Port=4
  theta_SG_D_1_out : Outport  Port=5
  wires:
  d_Px_1_SG_D_1_block/1(Blockout_d_Px_1_SG_D_1_e6c1c) -> Px_1_SG_D_1/1
  V_f_SG_D_1/1 -> d_V_f_SG_D_1_block/14(State_V_f_SG_D_1_83a86), d_E_fd_SG_D_1_block/2(State_V_f_SG_D_1_13267)
  psi_kq_SG_D_1/1 -> d_psi_q_SG_D_1_block/2(State_psi_kq_SG_D_1_bac7c), d_psi_gq_SG_D_1_block/3(State_psi_kq_SG_D_1_8f72b), d_psi_gq_SG_D_1_block/5(State_psi_kq_SG_D_1_97d2b), d_psi_kq_SG_D_1_block/4(State_psi_kq_SG_D_1_b0ad3), d_w_SG_D_1_block/5(State_psi_kq_SG_D_1_d2252), d_V_f_SG_D_1_block/10(State_psi_kq_SG_D_1_39648), d_psi_kq_SG_D_1_block/2(State_psi_kq_SG_D_1_f7f57), i_d_SG_D_1_block/2(State_psi_kq_SG_D_1_5abe0), i_q_SG_D_1_block/2(State_psi_kq_SG_D_1_4e43a), d_psi_gq_SG_D_1_block/8(State_psi_kq_SG_D_1_c6065), T_e_SG_D_1_block/3(State_psi_kq_SG_D_1_ea1db)
  w_SG_D_1_out_block/1(Blockout_w_SG_D_1_out_92872) -> w_SG_D_1_out/1
  d_theta_SG_D_1_block/1(Blockout_d_theta_SG_D_1_0d12b) -> theta_SG_D_1/1
  w_SG_D_1/1 -> d_psi_q_SG_D_1_block/9(State_w_SG_D_1_8f4a2), d_psi_d_SG_D_1_block/9(State_w_SG_D_1_53995), d_w_SG_D_1_block/1(State_w_SG_D_1_a377d), d_V_f_SG_D_1_block/8(State_w_SG_D_1_727da), d_V_f_SG_D_1_block/13(State_w_SG_D_1_0c346), d_theta_SG_D_1_block/1(State_w_SG_D_1_1349a), d_T_m_SG_D_1_block/1(State_w_SG_D_1_c2877), d_Px_1_SG_D_1_block/2(State_w_SG_D_1_7a36e), d_Px_3_SG_D_1_block/6(State_w_SG_D_1_55a2f), w_SG_D_1_out_block/1(State_w_SG_D_1_bec44), d_Px_2_SG_D_1_block/4(State_w_SG_D_1_5d530)
  d_Px_2_SG_D_1_block/1(Blockout_d_Px_2_SG_D_1_4e1cd) -> Px_2_SG_D_1/1
  d_Px_3_SG_D_1_block/1(Blockout_d_Px_3_SG_D_1_8cb1d) -> Px_3_SG_D_1/1
  d_T_m_SG_D_1_block/1(Blockout_d_T_m_SG_D_1_7bd94) -> T_m_SG_D_1/1
  psi_gq_SG_D_1/1 -> d_psi_q_SG_D_1_block/1(State_psi_gq_SG_D_1_c29fe), d_psi_gq_SG_D_1_block/2(State_psi_gq_SG_D_1_48022), d_psi_gq_SG_D_1_block/4(State_psi_gq_SG_D_1_3753d), d_V_f_SG_D_1_block/9(State_psi_gq_SG_D_1_8e6b5), d_psi_kq_SG_D_1_block/1(State_psi_gq_SG_D_1_5db4b), d_psi_gq_SG_D_1_block/1(State_psi_gq_SG_D_1_a269f), i_d_SG_D_1_block/1(State_psi_gq_SG_D_1_4d36f), d_psi_kq_SG_D_1_block/3(State_psi_gq_SG_D_1_83c8c), i_q_SG_D_1_block/1(State_psi_gq_SG_D_1_ff441), d_w_SG_D_1_block/4(State_psi_gq_SG_D_1_15c3e), d_psi_gq_SG_D_1_block/7(State_psi_gq_SG_D_1_de248), T_e_SG_D_1_block/2(State_psi_gq_SG_D_1_ab29c)
  psi_fd_SG_D_1/1 -> d_psi_fd_SG_D_1_block/2(State_psi_fd_SG_D_1_c9cc6), d_psi_fd_SG_D_1_block/4(State_psi_fd_SG_D_1_630cb), d_psi_fd_SG_D_1_block/7(State_psi_fd_SG_D_1_499fb), d_psi_fd_SG_D_1_block/10(State_psi_fd_SG_D_1_eb33a), d_psi_d_SG_D_1_block/3(State_psi_fd_SG_D_1_8eeeb), d_psi_1d_SG_D_1_block/5(State_psi_fd_SG_D_1_fd322), d_w_SG_D_1_block/10(State_psi_fd_SG_D_1_907bf), d_V_f_SG_D_1_block/6(State_psi_fd_SG_D_1_b9da0), d_psi_1d_SG_D_1_block/2(State_psi_fd_SG_D_1_6f731), i_d_SG_D_1_block/7(State_psi_fd_SG_D_1_52673), T_e_SG_D_1_block/8(State_psi_fd_SG_D_1_41c9f), i_q_SG_D_1_block/7(State_psi_fd_SG_D_1_5070a)
  Px_1_SG_D_1/1 -> d_Px_3_SG_D_1_block/4(State_Px_1_SG_D_1_e02b1), d_Px_2_SG_D_1_block/2(State_Px_1_SG_D_1_f11fa), d_Px_2_SG_D_1_block/3(State_Px_1_SG_D_1_b3d15), d_Px_1_SG_D_1_block/1(State_Px_1_SG_D_1_f6150), d_Px_3_SG_D_1_block/5(State_Px_1_SG_D_1_a6ed2)
  psi_q_SG_D_1/1 -> d_psi_d_SG_D_1_block/8(State_psi_q_SG_D_1_4f046), d_psi_q_SG_D_1_block/3(State_psi_q_SG_D_1_1d0c2), d_psi_gq_SG_D_1_block/6(State_psi_q_SG_D_1_55c4c), d_psi_gq_SG_D_1_block/9(State_psi_q_SG_D_1_b9c64), d_psi_kq_SG_D_1_block/5(State_psi_q_SG_D_1_db3ff), d_V_f_SG_D_1_block/7(State_psi_q_SG_D_1_faa61), d_w_SG_D_1_block/7(State_psi_q_SG_D_1_fc3d4), i_d_SG_D_1_block/3(State_psi_q_SG_D_1_b5d7f), d_w_SG_D_1_block/6(State_psi_q_SG_D_1_e0b00), T_e_SG_D_1_block/4(State_psi_q_SG_D_1_7ae8a), i_q_SG_D_1_block/3(State_psi_q_SG_D_1_65128), d_V_f_SG_D_1_block/11(State_psi_q_SG_D_1_bf0ee), T_e_SG_D_1_block/5(State_psi_q_SG_D_1_09903)
  d_E_fd_SG_D_1_block/1(Blockout_d_E_fd_SG_D_1_97a11) -> E_fd_SG_D_1/1
  psi_1d_SG_D_1/1 -> d_psi_fd_SG_D_1_block/5(State_psi_1d_SG_D_1_50752), d_psi_fd_SG_D_1_block/8(State_psi_1d_SG_D_1_2b625), d_psi_d_SG_D_1_block/1(State_psi_1d_SG_D_1_5fbb9), d_psi_1d_SG_D_1_block/1(State_psi_1d_SG_D_1_f4c7b), d_V_f_SG_D_1_block/4(State_psi_1d_SG_D_1_ff4f7), i_d_SG_D_1_block/5(State_psi_1d_SG_D_1_a973f), d_psi_fd_SG_D_1_block/3(State_psi_1d_SG_D_1_4b3bf), d_w_SG_D_1_block/8(State_psi_1d_SG_D_1_fbdce), i_q_SG_D_1_block/5(State_psi_1d_SG_D_1_b398b), d_psi_1d_SG_D_1_block/3(State_psi_1d_SG_D_1_bb128), T_e_SG_D_1_block/6(State_psi_1d_SG_D_1_b2d45)
  Px_2_SG_D_1/1 -> d_Px_2_SG_D_1_block/1(State_Px_2_SG_D_1_48e57), d_Px_3_SG_D_1_block/2(State_Px_2_SG_D_1_f2fa6), d_Px_3_SG_D_1_block/3(State_Px_2_SG_D_1_adf7b)
  theta_SG_D_1/1 -> d_psi_d_SG_D_1_block/5(State_theta_SG_D_1_4bc24), d_psi_d_SG_D_1_block/7(State_theta_SG_D_1_7b3a3), d_psi_q_SG_D_1_block/7(State_theta_SG_D_1_fb557), i_d_SG_D_1_block/4(State_theta_SG_D_1_47360), i_d_SG_D_1_block/8(State_theta_SG_D_1_0c5f1), d_psi_q_SG_D_1_block/5(State_theta_SG_D_1_d73f5), i_q_SG_D_1_block/4(State_theta_SG_D_1_2a693), i_q_SG_D_1_block/8(State_theta_SG_D_1_2605c), theta_SG_D_1_out_block/1(State_theta_SG_D_1_08b1b)
  v_d_SG_D_1/1 -> d_psi_d_SG_D_1_block/4(Input_v_d_SG_D_1_00b58), d_psi_q_SG_D_1_block/4(Input_v_d_SG_D_1_f7fec)
  v_q_SG_D_1/1 -> d_psi_d_SG_D_1_block/6(Input_v_q_SG_D_1_54b58), d_psi_q_SG_D_1_block/6(Input_v_q_SG_D_1_145b1)
  psi_d_SG_D_1/1 -> d_psi_fd_SG_D_1_block/6(State_psi_d_SG_D_1_74e73), d_psi_fd_SG_D_1_block/9(State_psi_d_SG_D_1_13107), d_psi_q_SG_D_1_block/8(State_psi_d_SG_D_1_00025), d_psi_1d_SG_D_1_block/4(State_psi_d_SG_D_1_52913), d_V_f_SG_D_1_block/5(State_psi_d_SG_D_1_8ec21), d_w_SG_D_1_block/3(State_psi_d_SG_D_1_23516), d_psi_d_SG_D_1_block/2(State_psi_d_SG_D_1_7394f), d_V_f_SG_D_1_block/12(State_psi_d_SG_D_1_565b7), i_q_SG_D_1_block/6(State_psi_d_SG_D_1_79e1a), d_w_SG_D_1_block/9(State_psi_d_SG_D_1_9e7e6), T_e_SG_D_1_block/1(State_psi_d_SG_D_1_20e40), i_d_SG_D_1_block/6(State_psi_d_SG_D_1_2da12), T_e_SG_D_1_block/7(State_psi_d_SG_D_1_5ffcd)
  T_m_SG_D_1/1 -> d_T_m_SG_D_1_block/2(State_T_m_SG_D_1_3f3eb), d_w_SG_D_1_block/2(State_T_m_SG_D_1_e54f4)
  d_R_f_SG_D_1_block/1(Blockout_d_R_f_SG_D_1_76ad3) -> R_f_SG_D_1/1
  i_q_SG_D_1_block/1(Blockout_i_q_SG_D_1_39ddb) -> i_q_SG_D_1/1
  d_V_f_SG_D_1_block/1(Blockout_d_V_f_SG_D_1_c02f4) -> V_f_SG_D_1/1
  i_d_SG_D_1_block/1(Blockout_i_d_SG_D_1_13e50) -> i_d_SG_D_1/1
  theta_SG_D_1_out_block/1(Blockout_theta_SG_D_1_out_85d64) -> theta_SG_D_1_out/1
  d_psi_gq_SG_D_1_block/1(Blockout_d_psi_gq_SG_D_1_d02c6) -> psi_gq_SG_D_1/1
  d_psi_1d_SG_D_1_block/1(Blockout_d_psi_1d_SG_D_1_8846c) -> psi_1d_SG_D_1/1
  d_psi_d_SG_D_1_block/1(Blockout_d_psi_d_SG_D_1_c980b) -> psi_d_SG_D_1/1
  d_psi_q_SG_D_1_block/1(Blockout_d_psi_q_SG_D_1_1eeca) -> psi_q_SG_D_1/1
  d_psi_kq_SG_D_1_block/1(Blockout_d_psi_kq_SG_D_1_8a28d) -> psi_kq_SG_D_1/1
  T_e_SG_D_1_block/1(Blockout_T_e_SG_D_1_92784) -> T_e_SG_D_1/1
  d_w_SG_D_1_block/1(Blockout_d_w_SG_D_1_13572) -> w_SG_D_1/1
  Px_3_SG_D_1/1 -> d_V_f_SG_D_1_block/3(State_Px_3_SG_D_1_9299b), d_Px_3_SG_D_1_block/1(State_Px_3_SG_D_1_4be19)
  R_f_SG_D_1/1 -> d_V_f_SG_D_1_block/2(State_R_f_SG_D_1_08feb), d_R_f_SG_D_1_block/2(State_R_f_SG_D_1_00ad4)
  E_fd_SG_D_1/1 -> d_R_f_SG_D_1_block/1(State_E_fd_SG_D_1_eb437), d_E_fd_SG_D_1_block/1(State_E_fd_SG_D_1_abc9a), d_V_f_SG_D_1_block/1(State_E_fd_SG_D_1_92169), d_psi_fd_SG_D_1_block/1(State_E_fd_SG_D_1_f3910)
  d_psi_fd_SG_D_1_block/1(Blockout_d_psi_fd_SG_D_1_b270d) -> psi_fd_SG_D_1/1
